simulink model "KTH_pedestrian_autoware_light_cs"  (R2019a)
settings: Solver=ode5  StartTime=0.0  StopTime=inf  FixedStep=1/20  RelTol=1e-3
PreLoadFcn:
  | mbxruntime.callbacks.PreLoadFcn(bdroot);
PostLoadFcn:
  | mbxruntime.callbacks.PostLoadFcn(bdroot);
InitFcn:
  | mbxruntime.callbacks.InitFcn(bdroot);
StartFcn:
  | mbxruntime.callbacks.StartFcn(bdroot);
StopFcn:
  | mbxruntime.callbacks.StopFcn(bdroot);
model workspace: external: MAT-File .\KTH_pedestrian_autoware_light_cs_hws.mat (data not in the file)
undefined symbols (not defined in the file or in its folder): DiscIntNeverNeededParam, KTH_pedestrian_autoware_light_cs_02ac950ed1db34ed, KTH_pedestrian_autoware_light_cs_05d7c050840f08db, KTH_pedestrian_autoware_light_cs_0ac3d38ce01e323f, KTH_pedestrian_autoware_light_cs_1214d37425b96e35, KTH_pedestrian_autoware_light_cs_2826e94662b29978, KTH_pedestrian_autoware_light_cs_284990f0f6de4093, KTH_pedestrian_autoware_light_cs_2ceb80ac95efe639, KTH_pedestrian_autoware_light_cs_5a38d8f46f118122, KTH_pedestrian_autoware_light_cs_6a647bfa7761b210, KTH_pedestrian_autoware_light_cs_790d47fa8c779a57, KTH_pedestrian_autoware_light_cs_7e2644aa1be91b53, KTH_pedestrian_autoware_light_cs_7f1596adbf6cd625, KTH_pedestrian_autoware_light_cs_8d332c892ff4a2b3, KTH_pedestrian_autoware_light_cs_a7eac5b1261ff56b, KTH_pedestrian_autoware_light_cs_b4a916664d8e8a9c, KTH_pedestrian_autoware_light_cs_ece26882e18d2248, KTH_pedestrian_autoware_light_cs_fb19b2cd0788cd5c, KTH_pedestrian_autoware_light_cs_fbb215df62dd156c, mbxruntime, tabledata, X, Y, Z
libraries: adeye_lib x16, PreScanSimulinkLibrary x6, robotlib x2, PreScanUsefulBlocks x1, simulink x1
(part 2 of 3)

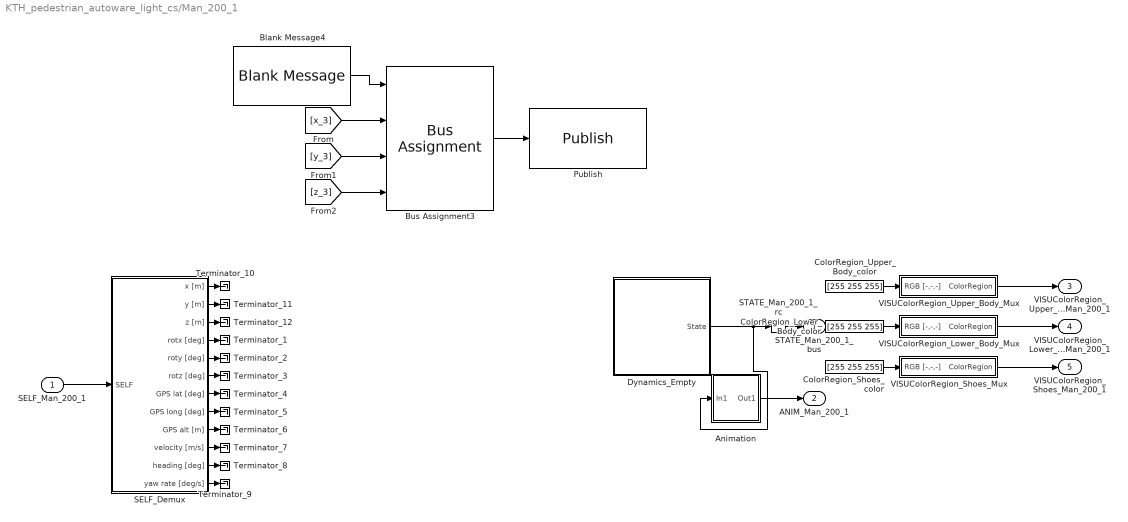
== system KTH_pedestrian_autoware_light_cs/Man_200_1 ==
  SELF_Man_200_1 : Inport  Tag=inport/SelfPort  OutDataTypeStr=Bus: PRESCAN_SELFSENSORDATA  PortDimensions=1  SampleTime=1/20  BusOutputAsStruct=on
  Animation : Subsystem  Tag=WalkingHumanAnimation  mask(Prescan Conversion Block: Walking Human Animation){TimeStep=1/20}
      mask prompts: TimeStep "Auto-Assigned: Upload Period [s]"
      mask help: The Walking Human Animation block converts the State signal of a human into signals to properly control the animation.
      mask Help: eval('openHelp(239)');
      mask Display: image(imread('HumanAnimated.jpg'))
  Blank Message4 : robotlib/Blank Message  messageClass=Message  entityType=geometry_msgs/Point  messageType=geometry_msgs/Point  SampleTime=inf
      settings: SourceProductBaseCode=RO
  Bus Assignment3 : BusAssignment  AssignedSignals=X,Y,Z
  ColorRegion_Lower_Body_color : Constant  Tag=VisuLightConst  Value=[255 255 255]
  ColorRegion_Shoes_color : Constant  Tag=VisuLightConst  Value=[255 255 255]
  ColorRegion_Upper_Body_color : Constant  Tag=VisuLightConst  Value=[255 255 255]
  Dynamics_Empty : Subsystem  Tag=Dynamics_Empty
      mask Help: eval('openHelp(202)')
      mask Display: port_label('output', 1, 'State');text(0,0,' Empty\n')
  Publish : robotlib/Publish  topicSource=Specify your own  topic=/simulink/pedestrian_pose  messageType=geometry_msgs/Point  messageQueueLength=1
      settings: SourceProductBaseCode=RO
  SELF_Demux : Subsystem  Tag=demux/SelfPort  mask(PreScan Demux Block:){}
      mask help:
      | The SELF port shows (state) information of the actor itself. The outputs are position in the experiment's axis system and the GPS coordinates, and the object's absolute velocity and compass heading.
      |
      | For more information, please click Help.
      settings: DeleteFcn=PreScanBlockDeleteFcn;
      mask Help: eval('openHelp(462)')
      mask Display:
      | port_label('output',1,'x [m]')
      | port_label('output',2,'y [m]')
      | port_label('output',3,'z [m]','texmode','on')
      | port_label('output',4,'Rotx [deg]','texmode','on')
      | port_label('output',5,'Roty [deg]','texmode','on')
      | port_label('output',6,'Rotz [deg]','texmode','on')
      | port_label('output',7,'GPS lat [deg]','texmode','on')
      | port_label('output',8,'GPS long [deg]','texmode','on')
      | port_label('output',9,'GPS alt [m]','texmode','on')
      | port_label('output',10,'Velocity [m/s]')
      | port_label('output',11,'Heading [deg]')
      | port_label('output',12,'Yaw rate [deg/s]')
  STATE_Man_200_1_rc : RateTransition  Tag=mux_rc/StatePort  OutPortSampleTimeOpt=Inherit
  Terminator_{1..12} (12 alike) : Terminator
  VISUColorRegion_Lower_Body_Mux : Subsystem  Tag=mux/MuxColorRegion  LoadFcn=load PrescanColorData  mask(PreScan User Interface: VisuTextureColor){}
      mask help:
      | The VisuTextureColor block provides a way to adapt the color of a vehicle.
      |
      | For more information, please click Help.
      settings: DeleteFcn=PreScanBlockDeleteFcn;
      mask Help: eval('openHelp(230)')
  VISUColorRegion_Shoes_Mux : Subsystem  Tag=mux/MuxColorRegion  LoadFcn=load PrescanColorData  mask(PreScan User Interface: VisuTextureColor){}
      mask help:
      | The VisuTextureColor block provides a way to adapt the color of a vehicle.
      |
      | For more information, please click Help.
      settings: DeleteFcn=PreScanBlockDeleteFcn;
      mask Help: eval('openHelp(230)')
  VISUColorRegion_Upper_Body_Mux : Subsystem  Tag=mux/MuxColorRegion  LoadFcn=load PrescanColorData  mask(PreScan User Interface: VisuTextureColor){}
      mask help:
      | The VisuTextureColor block provides a way to adapt the color of a vehicle.
      |
      | For more information, please click Help.
      settings: DeleteFcn=PreScanBlockDeleteFcn;
      mask Help: eval('openHelp(230)')
  STATE_Man_200_1_bus : Outport  Tag=outport/StatePort  OutDataTypeStr=Bus: PRESCAN_STATEACTUATORDATA  PortDimensions=1  SampleTime=1/20
  ANIM_Man_200_1 : Outport  Tag=outport/AnimationOutport  Port=2  OutDataTypeStr=Bus: PRESCAN_ANIMACTUATORDATA  PortDimensions=1  SampleTime=1/20
  VISUColorRegion_Upper_Body_Man_200_1 : Outport  Tag=outport/ColorRegion  Port=3  OutDataTypeStr=Bus: PRESCAN_COLOR_DATA  PortDimensions=1  SampleTime=1/20
  VISUColorRegion_Lower_Body_Man_200_1 : Outport  Tag=outport/ColorRegion  Port=4  OutDataTypeStr=Bus: PRESCAN_COLOR_DATA  PortDimensions=1  SampleTime=1/20
  VISUColorRegion_Shoes_Man_200_1 : Outport  Tag=outport/ColorRegion  Port=5  OutDataTypeStr=Bus: PRESCAN_COLOR_DATA  PortDimensions=1  SampleTime=1/20
  wires:
  Bus Assignment3/1 -> Publish/1
  Blank Message4/1 -> Bus Assignment3/1
  STATE_Man_200_1_rc/1 -> STATE_Man_200_1_bus/1
  Animation/1(Out1) -> ANIM_Man_200_1/1
  SELF_Man_200_1/1 -> SELF_Demux/1(SELF)
  VISUColorRegion_Upper_Body_Mux/1(ColorRegion) -> VISUColorRegion_Upper_Body_Man_200_1/1
  ColorRegion_Upper_Body_color/1 -> VISUColorRegion_Upper_Body_Mux/1(RGB [-,-,-])
  VISUColorRegion_Lower_Body_Mux/1(ColorRegion) -> VISUColorRegion_Lower_Body_Man_200_1/1
  ColorRegion_Lower_Body_color/1 -> VISUColorRegion_Lower_Body_Mux/1(RGB [-,-,-])
  VISUColorRegion_Shoes_Mux/1(ColorRegion) -> VISUColorRegion_Shoes_Man_200_1/1
  ColorRegion_Shoes_color/1 -> VISUColorRegion_Shoes_Mux/1(RGB [-,-,-])
  Dynamics_Empty/1(State) -> STATE_Man_200_1_rc/1, Animation/1(In1)
  SELF_Demux/4(rotx [deg]) -> Terminator_1/1
  SELF_Demux/5(roty [deg]) -> Terminator_2/1
  SELF_Demux/6(rotz [deg]) -> Terminator_3/1
  SELF_Demux/7(GPS lat [deg]) -> Terminator_4/1
  SELF_Demux/8(GPS long [deg]) -> Terminator_5/1
  SELF_Demux/9(GPS alt [m]) -> Terminator_6/1
  SELF_Demux/10(velocity [m/s]) -> Terminator_7/1
  SELF_Demux/11(heading [deg]) -> Terminator_8/1
  SELF_Demux/12(yaw rate [deg/s]) -> Terminator_9/1
  SELF_Demux/1(x [m]) -> Terminator_10/1
  SELF_Demux/2(y [m]) -> Terminator_11/1
  SELF_Demux/3(z [m]) -> Terminator_12/1
  [x_3] -> Bus Assignment3/2
  [y_3] -> Bus Assignment3/3
  [z_3] -> Bus Assignment3/4

== system KTH_pedestrian_autoware_light_cs/PointCloudSensor_1 ==
  Sensor : S-Function  FunctionName=sfun_PCS  Parameters=sensorID, dataWidth, dataHeight, numChannels, dataType, timestep  SFunctionDeploymentMode=off  EnableBusSupport=off  mask(PreScan Source Block: Point Cloud Sensor){sensorID=9052, dataWidth=16, dataHeight=900, numChannels=4, dataType=0, timestep=1/20}
      mask prompts: sensorID "Sensor ID"; dataWidth "Data Width"; dataHeight "Data Height"; numChannels "Channel Count"; dataType "Data Type"; timestep "MATLAB timestep:"
      mask help: The Point Cloud Sensor provides XYZ positions relative to the sensor
      mask Help: eval('openHelp(6400)')
      mask Display: image(imread('PointCloudSensorSL.png'))
  PointCloudSensor_1 : Outport  Tag=outport/PointCloudInport  OutDataTypeStr=single  SampleTime=1/20
  wires:
  Sensor/1 -> PointCloudSensor_1/1

== system KTH_pedestrian_autoware_light_cs/PointCloudSensor_2 ==
  Sensor : S-Function  FunctionName=sfun_PCS  Parameters=sensorID, dataWidth, dataHeight, numChannels, dataType, timestep  SFunctionDeploymentMode=off  EnableBusSupport=off  mask(PreScan Source Block: Point Cloud Sensor){sensorID=9053, dataWidth=16, dataHeight=900, numChannels=4, dataType=0, timestep=1/20}
      mask prompts: sensorID "Sensor ID"; dataWidth "Data Width"; dataHeight "Data Height"; numChannels "Channel Count"; dataType "Data Type"; timestep "MATLAB timestep:"
      mask help: The Point Cloud Sensor provides XYZ positions relative to the sensor
      mask Help: eval('openHelp(6400)')
      mask Display: image(imread('PointCloudSensorSL.png'))
  PointCloudSensor_2 : Outport  Tag=outport/PointCloudInport  OutDataTypeStr=single  SampleTime=1/20
  wires:
  Sensor/1 -> PointCloudSensor_2/1

== system KTH_pedestrian_autoware_light_cs/PointCloudSensor_3 ==
  Sensor : S-Function  FunctionName=sfun_PCS  Parameters=sensorID, dataWidth, dataHeight, numChannels, dataType, timestep  SFunctionDeploymentMode=off  EnableBusSupport=off  mask(PreScan Source Block: Point Cloud Sensor){sensorID=9054, dataWidth=16, dataHeight=900, numChannels=4, dataType=0, timestep=1/20}
      mask prompts: sensorID "Sensor ID"; dataWidth "Data Width"; dataHeight "Data Height"; numChannels "Channel Count"; dataType "Data Type"; timestep "MATLAB timestep:"
      mask help: The Point Cloud Sensor provides XYZ positions relative to the sensor
      mask Help: eval('openHelp(6400)')
      mask Display: image(imread('PointCloudSensorSL.png'))
  PointCloudSensor_3 : Outport  Tag=outport/PointCloudInport  OutDataTypeStr=single  SampleTime=1/20
  wires:
  Sensor/1 -> PointCloudSensor_3/1

== system KTH_pedestrian_autoware_light_cs/PointCloudSensor_4 ==
  Sensor : S-Function  FunctionName=sfun_PCS  Parameters=sensorID, dataWidth, dataHeight, numChannels, dataType, timestep  SFunctionDeploymentMode=off  EnableBusSupport=off  mask(PreScan Source Block: Point Cloud Sensor){sensorID=9055, dataWidth=16, dataHeight=900, numChannels=4, dataType=0, timestep=1/20}
      mask prompts: sensorID "Sensor ID"; dataWidth "Data Width"; dataHeight "Data Height"; numChannels "Channel Count"; dataType "Data Type"; timestep "MATLAB timestep:"
      mask help: The Point Cloud Sensor provides XYZ positions relative to the sensor
      mask Help: eval('openHelp(6400)')
      mask Display: image(imread('PointCloudSensorSL.png'))
  PointCloudSensor_4 : Outport  Tag=outport/PointCloudInport  OutDataTypeStr=single  SampleTime=1/20
  wires:
  Sensor/1 -> PointCloudSensor_4/1

== system KTH_pedestrian_autoware_light_cs/PreScanTerminator ==
  Terminator : Terminator
  sfun_Terminator : S-Function  FunctionName=sfun_Terminator  Parameters=SampleTime  SFunctionDeploymentMode=off  EnableBusSupport=off  mask(Legacy Function){SFunctionSpec=void prescan_terminator_outputFcn(void ** work1, PRESCAN_TERMINATORDATA y1[1]), SampleTime=TimeStep, ShowSpec=on}
      mask prompts: SampleTime "Sample time (-1 for inherited):"; ShowSpec "Display function specification"
      mask help:
      | This block allows you to call the legacy functions specified by the following Legacy Code Tool definition:
      | def.SFunctionName = 'sfun_Terminator';
      | def.OutputFcnSpec = 'void prescan_terminator_outputFcn(void ** work1, PRESCAN_TERMINATORDATA y1[1])';
      | def.StartFcnSpec = 'void prescan_terminator_startFcn(void ** work1)';
      | def.TerminateFcnSpec = 'void prescan_terminator_terminateFcn(void ** work1)';
      | def.HeaderFiles = {'prescan_terminator_data.h'};
      | def.HostLibFiles = {'sensorinterfaced.lib'};
      | def.IncPaths = {'src', 'C:\prescandev\vislibrary\vis\..\pimp\include\sensors\InterfaceRTW'};
      | def.SrcPaths = {'src'};
      | def.LibPaths = {'C:\\prescandev\\vislibrary_build\lib'};
      | def.SampleTime = 'parameterized';
      | def.Options.language = 'C';
      mask Help: <p>This block was generated automatically by the Legacy Code Tool. For detailed help on this tool, call<a href="matlab:legacy_code('help')"> legacy_code('help')</a>.</p>
      mask Callback ShowSpec:
      | if strcmp(get_param(gcbh, 'ShowSpec'), 'on')
      |   set_param(gcbh, 'MaskDisplay', sprintf('fprintf(''%s'');', get_param(gcbh, 'SFunctionSpec')));
      | else
      |   set_param(gcbh, 'MaskDisplay', sprintf('fprintf(''%s'');', get_param(gcbh, 'FunctionName')));
      | end
      mask Display: fprintf('void prescan_terminator_outputFcn(void ** work1, PRESCAN_TERMINATORDATA y1[1])');
  wires:
  sfun_Terminator/1 -> Terminator/1

== system KTH_pedestrian_autoware_light_cs/Radar_1 ==
  Sensor : S-Function  FunctionName=sfun_Radar  Parameters=sensorID, detectableObjects, timestep  SFunctionDeploymentMode=off  EnableBusSupport=off  mask(PreScan Source Block: Radar Sensor){sensorID=21907, detectableObjects=7, timestep=1/20}
      mask prompts: sensorID "Sensor ID"; detectableObjects "Max detectable objects:"; timestep "MATLAB timestep:"
      mask help:
      | The Radar Sensor is a detailed sensor based on a physical radar
      | model that includes Antenna GAIN Maps (AGM) and atmospheric
      | attenuation.
      |
      | For more information, please click Help.
      mask Help: eval('openHelp(1464)')
      mask Display: image(imread('Radar.png'))
  Radar_1 : Outport  Tag=outport/Radar  OutDataTypeStr=Bus: PRESCAN_SCANNERSENSOR_MESSAGE  PortDimensions=7  SampleTime=1/20
  wires:
  Sensor/1 -> Radar_1/1

== system KTH_pedestrian_autoware_light_cs/SELF_BMW_X5_SUV_1 ==
  Sensor : S-Function  FunctionName=sfun_SelfSensor  Parameters=UniqueID, TimeStep  SFunctionDeploymentMode=off  EnableBusSupport=off  mask(PreScan Source Block: SELF){UniqueID=9040, TimeStep=1/20}
      mask prompts: UniqueID "Auto-Assigned: Unique ID"; TimeStep "Auto-Assigned: Upload Period [s]"
      mask help:
      | The SELF port shows (state) information of the actor itself. The outputs are position in the experiment's axis system and the GPS coordinates, and the object's absolute velocity and compass heading.
      |
      | For more information, please click Help.
      mask Help: eval('openHelp(462)')
      mask Display: image(imread('GPS.png'))
  SELF_BMW_X5_SUV_1 : Outport  Tag=outport/SelfPort  OutDataTypeStr=Bus: PRESCAN_SELFSENSORDATA  PortDimensions=1  SampleTime=1/20
  wires:
  Sensor/1 -> SELF_BMW_X5_SUV_1/1

== system KTH_pedestrian_autoware_light_cs/SELF_KTH_3D_1 ==
  Sensor : S-Function  FunctionName=sfun_SelfSensor  Parameters=UniqueID, TimeStep  SFunctionDeploymentMode=off  EnableBusSupport=off  mask(PreScan Source Block: SELF){UniqueID=14987, TimeStep=1/20}
      mask prompts: UniqueID "Auto-Assigned: Unique ID"; TimeStep "Auto-Assigned: Upload Period [s]"
      mask help:
      | The SELF port shows (state) information of the actor itself. The outputs are position in the experiment's axis system and the GPS coordinates, and the object's absolute velocity and compass heading.
      |
      | For more information, please click Help.
      mask Help: eval('openHelp(462)')
      mask Display: image(imread('GPS.png'))
  SELF_KTH_3D_1 : Outport  Tag=outport/SelfPort  OutDataTypeStr=Bus: PRESCAN_SELFSENSORDATA  PortDimensions=1  SampleTime=1/20
  wires:
  Sensor/1 -> SELF_KTH_3D_1/1

== system KTH_pedestrian_autoware_light_cs/SELF_Man_200_1 ==
  Sensor : S-Function  FunctionName=sfun_SelfSensor  Parameters=UniqueID, TimeStep  SFunctionDeploymentMode=off  EnableBusSupport=off  mask(PreScan Source Block: SELF){UniqueID=20104, TimeStep=1/20}
      mask prompts: UniqueID "Auto-Assigned: Unique ID"; TimeStep "Auto-Assigned: Upload Period [s]"
      mask help:
      | The SELF port shows (state) information of the actor itself. The outputs are position in the experiment's axis system and the GPS coordinates, and the object's absolute velocity and compass heading.
      |
      | For more information, please click Help.
      mask Help: eval('openHelp(462)')
      mask Display: image(imread('GPS.png'))
  SELF_Man_200_1 : Outport  Tag=outport/SelfPort  OutDataTypeStr=Bus: PRESCAN_SELFSENSORDATA  PortDimensions=1  SampleTime=1/20
  wires:
  Sensor/1 -> SELF_Man_200_1/1

== system KTH_pedestrian_autoware_light_cs/STATE_BMW_X5_SUV_1_bus ==
  STATE_BMW_X5_SUV_1_bus : Inport  Tag=inport/StatePort  OutDataTypeStr=Bus: PRESCAN_STATEACTUATORDATA  PortDimensions=1  SampleTime=1/20  BusOutputAsStruct=on
  Actuator : S-Function  FunctionName=sfun_StateActuator  Parameters=UniqueID, TimeStep  SFunctionDeploymentMode=off  EnableBusSupport=off  mask(PreScan Sink Block: State){UniqueID=9040, TimeStep=1/20}
      mask prompts: UniqueID "Auto-Assigned: Unique ID"; TimeStep "Auto-Assigned: Upload Period [s]"
      mask help:
      | The Actor State contains a vector signal of size (9x1), containing the following signals:
      |
      | -  Position    	(x,y,z)             	[m]
      | -  Velocity    	(vx,vy,vz)         	[m/s]
      | -  Angles       	(Roll, Pitch, Yaw)	[rad]
      |
      | The Actor state is defined in the global axis system.
      | The state is superponed on the Initial position defined in the GUI.
      |
      | For more information, please click Help.
      mask Help: eval('openHelp(222)')
      mask Display: image(imread('State.png'))
  wires:
  STATE_BMW_X5_SUV_1_bus/1 -> Actuator/1

== system KTH_pedestrian_autoware_light_cs/STATE_KTH_3D_1_bus ==
  STATE_KTH_3D_1_bus : Inport  Tag=inport/StatePort  OutDataTypeStr=Bus: PRESCAN_STATEACTUATORDATA  PortDimensions=1  SampleTime=1/20  BusOutputAsStruct=on
  Actuator : S-Function  FunctionName=sfun_StateActuator  Parameters=UniqueID, TimeStep  SFunctionDeploymentMode=off  EnableBusSupport=off  mask(PreScan Sink Block: State){UniqueID=14987, TimeStep=1/20}
      mask prompts: UniqueID "Auto-Assigned: Unique ID"; TimeStep "Auto-Assigned: Upload Period [s]"
      mask help:
      | The Actor State contains a vector signal of size (9x1), containing the following signals:
      |
      | -  Position    	(x,y,z)             	[m]
      | -  Velocity    	(vx,vy,vz)         	[m/s]
      | -  Angles       	(Roll, Pitch, Yaw)	[rad]
      |
      | The Actor state is defined in the global axis system.
      | The state is superponed on the Initial position defined in the GUI.
      |
      | For more information, please click Help.
      mask Help: eval('openHelp(222)')
      mask Display: image(imread('State.png'))
  wires:
  STATE_KTH_3D_1_bus/1 -> Actuator/1

== system KTH_pedestrian_autoware_light_cs/STATE_Man_200_1_bus ==
  STATE_Man_200_1_bus : Inport  Tag=inport/StatePort  OutDataTypeStr=Bus: PRESCAN_STATEACTUATORDATA  PortDimensions=1  SampleTime=1/20  BusOutputAsStruct=on
  Actuator : S-Function  FunctionName=sfun_StateActuator  Parameters=UniqueID, TimeStep  SFunctionDeploymentMode=off  EnableBusSupport=off  mask(PreScan Sink Block: State){UniqueID=20104, TimeStep=1/20}
      mask prompts: UniqueID "Auto-Assigned: Unique ID"; TimeStep "Auto-Assigned: Upload Period [s]"
      mask help:
      | The Actor State contains a vector signal of size (9x1), containing the following signals:
      |
      | -  Position    	(x,y,z)             	[m]
      | -  Velocity    	(vx,vy,vz)         	[m/s]
      | -  Angles       	(Roll, Pitch, Yaw)	[rad]
      |
      | The Actor state is defined in the global axis system.
      | The state is superponed on the Initial position defined in the GUI.
      |
      | For more information, please click Help.
      mask Help: eval('openHelp(222)')
      mask Display: image(imread('State.png'))
  wires:
  STATE_Man_200_1_bus/1 -> Actuator/1

== system KTH_pedestrian_autoware_light_cs/ScenarioEngine ==
  Clock : Clock
  sfun_ScenarioEngine : S-Function  FunctionName=sfun_ScenarioEngine  Parameters=TimeStep  SFunctionDeploymentMode=off  EnableBusSupport=off
  wires:
  Clock/1 -> sfun_ScenarioEngine/1

== system KTH_pedestrian_autoware_light_cs/Synchronizer ==
  Bus Selector1 : BusSelector  OutputSignals=FederateStopped
  Stop Simulation : Stop
  sfun_Synchronizer : S-Function  FunctionName=sfun_Synchronizer  Parameters=SampleTime  SFunctionDeploymentMode=off  EnableBusSupport=off  mask(Legacy Function){SFunctionSpec=void prescan_synchronizer_outputFcn(void ** work1, PRESCAN_SYNCHRONIZEDATA y1[1]), SampleTime=TimeStep, ShowSpec=on}
      mask prompts: SampleTime "Sample time (-1 for inherited):"; ShowSpec "Display function specification"
      mask help:
      | This block allows you to call the legacy functions specified by the following Legacy Code Tool definition:
      | def.SFunctionName = 'sfun_Synchronizer';
      | def.OutputFcnSpec = 'void prescan_synchronizer_outputFcn(void ** work1, PRESCAN_SYNCHRONIZEDATA y1[1])';
      | def.StartFcnSpec = 'void prescan_synchronizer_startFcn(void ** work1)';
      | def.TerminateFcnSpec = 'void prescan_synchronizer_terminateFcn(void ** work1)';
      | def.HeaderFiles = {'prescan_synchronizer_data.h'};
      | def.HostLibFiles = {'sensorinterfaced.lib'};
      | def.IncPaths = {'src', 'C:\prescandev\vislibrary\vis\..\pimp\include\sensors\InterfaceRTW'};
      | def.SrcPaths = {'src'};
      | def.LibPaths = {'C:\\prescandev\\vislibrary_build\lib'};
      | def.SampleTime = 'parameterized';
      | def.Options.language = 'C';
      mask Help: <p>This block was generated automatically by the Legacy Code Tool. For detailed help on this tool, call<a href="matlab:legacy_code('help')"> legacy_code('help')</a>.</p>
      mask Callback ShowSpec:
      | if strcmp(get_param(gcbh, 'ShowSpec'), 'on')
      |   set_param(gcbh, 'MaskDisplay', sprintf('fprintf(''%s'');', get_param(gcbh, 'SFunctionSpec')));
      | else
      |   set_param(gcbh, 'MaskDisplay', sprintf('fprintf(''%s'');', get_param(gcbh, 'FunctionName')));
      | end
      mask Display: fprintf('void prescan_synchronizer_outputFcn(void ** work1, PRESCAN_SYNCHRONIZEDATA y1[1])');
  wires:
  Bus Selector1/1 -> Stop Simulation/1  "<FederateStopped>"
  sfun_Synchronizer/1 -> Bus Selector1/1

== system KTH_pedestrian_autoware_light_cs/VISUColorRegion_Lower_Body_Man_200_1 ==
  VISUColorRegion_Lower_Body_Man_200_1 : Inport  Tag=inport/ColorRegion  OutDataTypeStr=Bus: PRESCAN_COLOR_DATA  PortDimensions=1  SampleTime=1/20  BusOutputAsStruct=on
  Actuator : S-Function  FunctionName=sfun_ColorActuator  Parameters=mbxruntime.parameters.convert(UniqueID), mbxruntime.parameters.convert(WorldModelSubPath),tabledata, TimeStep  SFunctionDeploymentMode=off  EnableBusSupport=off  mask(PreScan Sink Block: VisuTextureColor){UniqueID=20104, WorldModelSubPath=/recolorRegion:name=Lower Body/targetColor, TimeStep=1/20}
      mask prompts: UniqueID "Parent Unique Identifier (auto-generated)"; WorldModelSubPath "WM SubPath(auto-generated)"; TimeStep "Simulink time step"
      mask help:
      | The VisuTextureColor block provides a way to adapt the color of a vehicle.
      |
      | For more information, please click Help.
      mask init:
      | [tabledata] = mbxruntime.parameters.table(UniqueID,WorldModelSubPath);
      mask Help: eval('openHelp(230)')
      mask Display: image(imread('TextureColor.png'))
  wires:
  VISUColorRegion_Lower_Body_Man_200_1/1 -> Actuator/1

== system KTH_pedestrian_autoware_light_cs/VISUColorRegion_Shoes_Man_200_1 ==
  VISUColorRegion_Shoes_Man_200_1 : Inport  Tag=inport/ColorRegion  OutDataTypeStr=Bus: PRESCAN_COLOR_DATA  PortDimensions=1  SampleTime=1/20  BusOutputAsStruct=on
  Actuator : S-Function  FunctionName=sfun_ColorActuator  Parameters=mbxruntime.parameters.convert(UniqueID), mbxruntime.parameters.convert(WorldModelSubPath),tabledata, TimeStep  SFunctionDeploymentMode=off  EnableBusSupport=off  mask(PreScan Sink Block: VisuTextureColor){UniqueID=20104, WorldModelSubPath=/recolorRegion:name=Shoes/targetColor, TimeStep=1/20}
      mask prompts: UniqueID "Parent Unique Identifier (auto-generated)"; WorldModelSubPath "WM SubPath(auto-generated)"; TimeStep "Simulink time step"
      mask help:
      | The VisuTextureColor block provides a way to adapt the color of a vehicle.
      |
      | For more information, please click Help.
      mask init:
      | [tabledata] = mbxruntime.parameters.table(UniqueID,WorldModelSubPath);
      mask Help: eval('openHelp(230)')
      mask Display: image(imread('TextureColor.png'))
  wires:
  VISUColorRegion_Shoes_Man_200_1/1 -> Actuator/1

== system KTH_pedestrian_autoware_light_cs/VISUColorRegion_Upper_Body_Man_200_1 ==
  VISUColorRegion_Upper_Body_Man_200_1 : Inport  Tag=inport/ColorRegion  OutDataTypeStr=Bus: PRESCAN_COLOR_DATA  PortDimensions=1  SampleTime=1/20  BusOutputAsStruct=on
  Actuator : S-Function  FunctionName=sfun_ColorActuator  Parameters=mbxruntime.parameters.convert(UniqueID), mbxruntime.parameters.convert(WorldModelSubPath),tabledata, TimeStep  SFunctionDeploymentMode=off  EnableBusSupport=off  mask(PreScan Sink Block: VisuTextureColor){UniqueID=20104, WorldModelSubPath=/recolorRegion:name=Upper Body/targetColor, TimeStep=1/20}
      mask prompts: UniqueID "Parent Unique Identifier (auto-generated)"; WorldModelSubPath "WM SubPath(auto-generated)"; TimeStep "Simulink time step"
      mask help:
      | The VisuTextureColor block provides a way to adapt the color of a vehicle.
      |
      | For more information, please click Help.
      mask init:
      | [tabledata] = mbxruntime.parameters.table(UniqueID,WorldModelSubPath);
      mask Help: eval('openHelp(230)')
      mask Display: image(imread('TextureColor.png'))
  wires:
  VISUColorRegion_Upper_Body_Man_200_1/1 -> Actuator/1

== system KTH_pedestrian_autoware_light_cs/BMW_X5_SUV_1/Camera_1_CM_Demux ==
  In1 : Inport
  Selector : Selector  NumberOfDimensions=2  InputPortWidth=3  IndexOptions=Index vector (dialog),Index vector (dialog)  Indices=-1,1:hres  OutputSizes=1,1
  Selector1 : Selector  NumberOfDimensions=2  InputPortWidth=3  IndexOptions=Index vector (dialog),Index vector (dialog)  Indices=-1,hres+1:hres*2  OutputSizes=1,1
  Selector2 : Selector  NumberOfDimensions=2  InputPortWidth=3  IndexOptions=Index vector (dialog),Index vector (dialog)  Indices=-1,hres*2+1:hres*3  OutputSizes=1,1
  R : Outport
  G : Outport  Port=2
  B : Outport  Port=3
  wires:
  In1/1 -> Selector1/1, Selector/1, Selector2/1
  Selector/1 -> R/1
  Selector1/1 -> G/1
  Selector2/1 -> B/1

== system KTH_pedestrian_autoware_light_cs/BMW_X5_SUV_1/Camera_2_CM_Demux ==
  In1 : Inport
  Selector : Selector  NumberOfDimensions=2  InputPortWidth=3  IndexOptions=Index vector (dialog),Index vector (dialog)  Indices=-1,1:hres  OutputSizes=1,1
  Selector1 : Selector  NumberOfDimensions=2  InputPortWidth=3  IndexOptions=Index vector (dialog),Index vector (dialog)  Indices=-1,hres+1:hres*2  OutputSizes=1,1
  Selector2 : Selector  NumberOfDimensions=2  InputPortWidth=3  IndexOptions=Index vector (dialog),Index vector (dialog)  Indices=-1,hres*2+1:hres*3  OutputSizes=1,1
  R : Outport
  G : Outport  Port=2
  B : Outport  Port=3
  wires:
  In1/1 -> Selector1/1, Selector/1, Selector2/1
  Selector/1 -> R/1
  Selector1/1 -> G/1
  Selector2/1 -> B/1

== system KTH_pedestrian_autoware_light_cs/BMW_X5_SUV_1/Camera_tl_CM_Demux ==
  In1 : Inport
  Selector : Selector  NumberOfDimensions=2  InputPortWidth=3  IndexOptions=Index vector (dialog),Index vector (dialog)  Indices=-1,1:hres  OutputSizes=1,1
  Selector1 : Selector  NumberOfDimensions=2  InputPortWidth=3  IndexOptions=Index vector (dialog),Index vector (dialog)  Indices=-1,hres+1:hres*2  OutputSizes=1,1
  Selector2 : Selector  NumberOfDimensions=2  InputPortWidth=3  IndexOptions=Index vector (dialog),Index vector (dialog)  Indices=-1,hres*2+1:hres*3  OutputSizes=1,1
  R : Outport
  G : Outport  Port=2
  B : Outport  Port=3
  wires:
  In1/1 -> Selector1/1, Selector/1, Selector2/1
  Selector/1 -> R/1
  Selector1/1 -> G/1
  Selector2/1 -> B/1

== system KTH_pedestrian_autoware_light_cs/BMW_X5_SUV_1/Dynamics_Empty ==
  note: For state mode 'Dynamic' positions
      | are not taken into account, as they
      | are computed by integrating velocity.
      | Click annotation for Help.
  Ground_{1..9} (9 alike) : Ground
  MuxState : Subsystem  Tag=mux/State  mask(Empty Dynamics State Block){positioningmode=on, TimeStep=1/20}
      mask prompts: positioningmode "Positioning Mode"; TimeStep "Auto Assigned: Time Step [s]"
      mask help:
      | Build the state of an actor based on user input.
      | The user can either use positioning mode or dynamics mode.
      | - When using positioning mode the position and orientation of the actor are set directly based on the input. Expected input is relative to the initial position and orientation of the actor. It's also possible to specify the velocity of the actor, though this input isn't used, only passed on.
      | - When using dynamics mode the position input is ignored. Expected input is velocity and orientation. The velocity is relative the current orientation of the actor, while orientation is relative to its initial orientation. The position of the actor is calculated based on the velocity and orientation given.
      settings: DeleteFcn=PreScanBlockDeleteFcn;
  STATE_BMW_X5_SUV_1 : Subsystem  Tag=mux/StatePort  Priority=0  LoadFcn=load PrescanStateActuatorData  mask(PreScan Sink Block: State){x0=KTH_pedestrian_autoware_light_cs_b4a916664d8e8a9c, y0=KTH_pedestrian_autoware_light_cs_1214d37425b96e35, z0=KTH_pedestrian_autoware_light_cs_2ceb80ac95efe639, Roll0=KTH_pedestrian_autoware_light_cs_7f1596adbf6cd625, Pitch0=KTH_pedestrian_autoware_light_cs_8d332c892ff4a2b3, Yaw0=KTH_pedestrian_autoware_light_cs_02ac950ed1db34ed, TimeStep=1/20}
      mask prompts: x0 "Ini x-position VEHICLE wrt GLOBAL axis system [m]"; y0 "Ini y-position VEHICLE wrt GLOBAL axis system [m]"; z0 "Ini z-position VEHICLE wrt GLOBAL axis system [m]"; Roll0 "Ini roll-angle BODY wrt VEHICLE axis system [deg]"; Pitch0 "Ini pitch-angle BODY wrt VEHICLE axis system [deg]"; Yaw0 "Ini yaw-angle VEHICLE wrt GLOBAL axis system [deg]"; TimeStep "Auto-Assigned: Upload Period [s]"
      mask help:
      | The Actor State contains a vector signal of size (9x1), containing the following signals:
      |
      | -  Position                  (x,y,z)                                     [m]
      | -  Velocity                  (vx,vy,vz)                               [m/s]
      | -  Angles                    (Roll, Pitch, Yaw)                   [rad]
      |
      | The Actor state is defined in the global axis system.
      | The state is superponed on the Initial position defined in the GUI.
      |
      | For more information, please click Help.
      settings: DeleteFcn=PreScanBlockDeleteFcn;
      mask Help: eval('openHelp(222)')
      mask Display: image(imread('State.png'))
  State : Outport  Tag=outport/StateOutport  SampleTime=1/20
  wires:
  MuxState/1(state) -> STATE_BMW_X5_SUV_1/1(State)
  STATE_BMW_X5_SUV_1/1(StateBus) -> State/1
  Ground_1/1 -> MuxState/1(x [m])
  Ground_2/1 -> MuxState/2(y [m])
  Ground_3/1 -> MuxState/3(z [m])
  Ground_4/1 -> MuxState/4(dx [m/s])
  Ground_5/1 -> MuxState/5(dy [m/s])
  Ground_6/1 -> MuxState/6(dz [m/s])
  Ground_7/1 -> MuxState/7(R [rad])
  Ground_8/1 -> MuxState/8(P [rad])
  Ground_9/1 -> MuxState/9(Y [rad])

== system KTH_pedestrian_autoware_light_cs/BMW_X5_SUV_1/PointCloudSensor_1_Angles_Demux ==
  In2 : Inport
  Selector : Selector  NumberOfDimensions=2  InputPortWidth=3  IndexOptions=Index vector (dialog),Index vector (dialog)  Indices=-1,offset+1:(offset+hres)  OutputSizes=1,1
  Selector1 : Selector  NumberOfDimensions=2  InputPortWidth=3  IndexOptions=Index vector (dialog),Index vector (dialog)  Indices=-1,(offset+hres+1):(offset+2*hres)  OutputSizes=1,1
  Theta : Outport
  Phi : Outport  Port=2
  wires:
  Selector1/1 -> Phi/1
  Selector/1 -> Theta/1
  In2/1 -> Selector/1, Selector1/1

== system KTH_pedestrian_autoware_light_cs/BMW_X5_SUV_1/PointCloudSensor_1_Intensity_Demux ==
  In1 : Inport
  Selector3 : Selector  NumberOfDimensions=2  InputPortWidth=3  IndexOptions=Index vector (dialog),Index vector (dialog)  Indices=-1,offset+1:(offset+hres)  OutputSizes=1,1
  Intensity : Outport
  wires:
  Selector3/1 -> Intensity/1
  In1/1 -> Selector3/1

== system KTH_pedestrian_autoware_light_cs/BMW_X5_SUV_1/PointCloudSensor_1_Range_Demux ==
  In1 : Inport
  Selector : Selector  NumberOfDimensions=2  InputPortWidth=3  IndexOptions=Index vector (dialog),Index vector (dialog)  Indices=-1,offset+1:(offset+hres)  OutputSizes=1,1
  Range : Outport
  wires:
  Selector/1 -> Range/1
  In1/1 -> Selector/1

== system KTH_pedestrian_autoware_light_cs/BMW_X5_SUV_1/PointCloudSensor_2_Angles_Demux ==
  In2 : Inport
  Selector : Selector  NumberOfDimensions=2  InputPortWidth=3  IndexOptions=Index vector (dialog),Index vector (dialog)  Indices=-1,offset+1:(offset+hres)  OutputSizes=1,1
  Selector1 : Selector  NumberOfDimensions=2  InputPortWidth=3  IndexOptions=Index vector (dialog),Index vector (dialog)  Indices=-1,(offset+hres+1):(offset+2*hres)  OutputSizes=1,1
  Theta : Outport
  Phi : Outport  Port=2
  wires:
  Selector1/1 -> Phi/1
  Selector/1 -> Theta/1
  In2/1 -> Selector/1, Selector1/1

== system KTH_pedestrian_autoware_light_cs/BMW_X5_SUV_1/PointCloudSensor_2_Intensity_Demux ==
  In1 : Inport
  Selector3 : Selector  NumberOfDimensions=2  InputPortWidth=3  IndexOptions=Index vector (dialog),Index vector (dialog)  Indices=-1,offset+1:(offset+hres)  OutputSizes=1,1
  Intensity : Outport
  wires:
  Selector3/1 -> Intensity/1
  In1/1 -> Selector3/1

== system KTH_pedestrian_autoware_light_cs/BMW_X5_SUV_1/PointCloudSensor_2_Range_Demux ==
  In1 : Inport
  Selector : Selector  NumberOfDimensions=2  InputPortWidth=3  IndexOptions=Index vector (dialog),Index vector (dialog)  Indices=-1,offset+1:(offset+hres)  OutputSizes=1,1
  Range : Outport
  wires:
  Selector/1 -> Range/1
  In1/1 -> Selector/1

== system KTH_pedestrian_autoware_light_cs/BMW_X5_SUV_1/PointCloudSensor_3_Angles_Demux ==
  In2 : Inport
  Selector : Selector  NumberOfDimensions=2  InputPortWidth=3  IndexOptions=Index vector (dialog),Index vector (dialog)  Indices=-1,offset+1:(offset+hres)  OutputSizes=1,1
  Selector1 : Selector  NumberOfDimensions=2  InputPortWidth=3  IndexOptions=Index vector (dialog),Index vector (dialog)  Indices=-1,(offset+hres+1):(offset+2*hres)  OutputSizes=1,1
  Theta : Outport
  Phi : Outport  Port=2
  wires:
  Selector1/1 -> Phi/1
  Selector/1 -> Theta/1
  In2/1 -> Selector/1, Selector1/1

== system KTH_pedestrian_autoware_light_cs/BMW_X5_SUV_1/PointCloudSensor_3_Intensity_Demux ==
  In1 : Inport
  Selector3 : Selector  NumberOfDimensions=2  InputPortWidth=3  IndexOptions=Index vector (dialog),Index vector (dialog)  Indices=-1,offset+1:(offset+hres)  OutputSizes=1,1
  Intensity : Outport
  wires:
  Selector3/1 -> Intensity/1
  In1/1 -> Selector3/1

== system KTH_pedestrian_autoware_light_cs/BMW_X5_SUV_1/PointCloudSensor_3_Range_Demux ==
  In1 : Inport
  Selector : Selector  NumberOfDimensions=2  InputPortWidth=3  IndexOptions=Index vector (dialog),Index vector (dialog)  Indices=-1,offset+1:(offset+hres)  OutputSizes=1,1
  Range : Outport
  wires:
  Selector/1 -> Range/1
  In1/1 -> Selector/1

== system KTH_pedestrian_autoware_light_cs/BMW_X5_SUV_1/PointCloudSensor_4_Angles_Demux ==
  In2 : Inport
  Selector : Selector  NumberOfDimensions=2  InputPortWidth=3  IndexOptions=Index vector (dialog),Index vector (dialog)  Indices=-1,offset+1:(offset+hres)  OutputSizes=1,1
  Selector1 : Selector  NumberOfDimensions=2  InputPortWidth=3  IndexOptions=Index vector (dialog),Index vector (dialog)  Indices=-1,(offset+hres+1):(offset+2*hres)  OutputSizes=1,1
  Theta : Outport
  Phi : Outport  Port=2
  wires:
  Selector1/1 -> Phi/1
  Selector/1 -> Theta/1
  In2/1 -> Selector/1, Selector1/1

== system KTH_pedestrian_autoware_light_cs/BMW_X5_SUV_1/PointCloudSensor_4_Intensity_Demux ==
  In1 : Inport
  Selector3 : Selector  NumberOfDimensions=2  InputPortWidth=3  IndexOptions=Index vector (dialog),Index vector (dialog)  Indices=-1,offset+1:(offset+hres)  OutputSizes=1,1
  Intensity : Outport
  wires:
  Selector3/1 -> Intensity/1
  In1/1 -> Selector3/1

== system KTH_pedestrian_autoware_light_cs/BMW_X5_SUV_1/PointCloudSensor_4_Range_Demux ==
  In1 : Inport
  Selector : Selector  NumberOfDimensions=2  InputPortWidth=3  IndexOptions=Index vector (dialog),Index vector (dialog)  Indices=-1,offset+1:(offset+hres)  OutputSizes=1,1
  Range : Outport
  wires:
  Selector/1 -> Range/1
  In1/1 -> Selector/1

== system KTH_pedestrian_autoware_light_cs/BMW_X5_SUV_1/Radar_1_Demux ==
  Radar : Inport
  Bus Selector1 : BusSelector  OutputSignals=ActiveBeamID[-],Range[m],DopplerVelocity[ms-1],DopplerVelocityX[ms-1],DopplerVelocityY[ms-1],DopplerVelocityZ[ms-1],Theta[deg],Phi[deg],TargetID[-],TargetTypeID[-],EnergyLoss[dB],Alpha[deg],Beta[deg]  OutputAsBus=on
  ScannerSensorLegacyBusConversion : PreScanUsefulBlocks/ScannerSensorLegacyBusConversion  MAXMESSAGES=MAXMESSAGES
  Radar Data : Outport
  wires:
  Bus Selector1/1 -> Radar Data/1
  ScannerSensorLegacyBusConversion/1 -> Bus Selector1/1
  Radar/1 -> ScannerSensorLegacyBusConversion/1

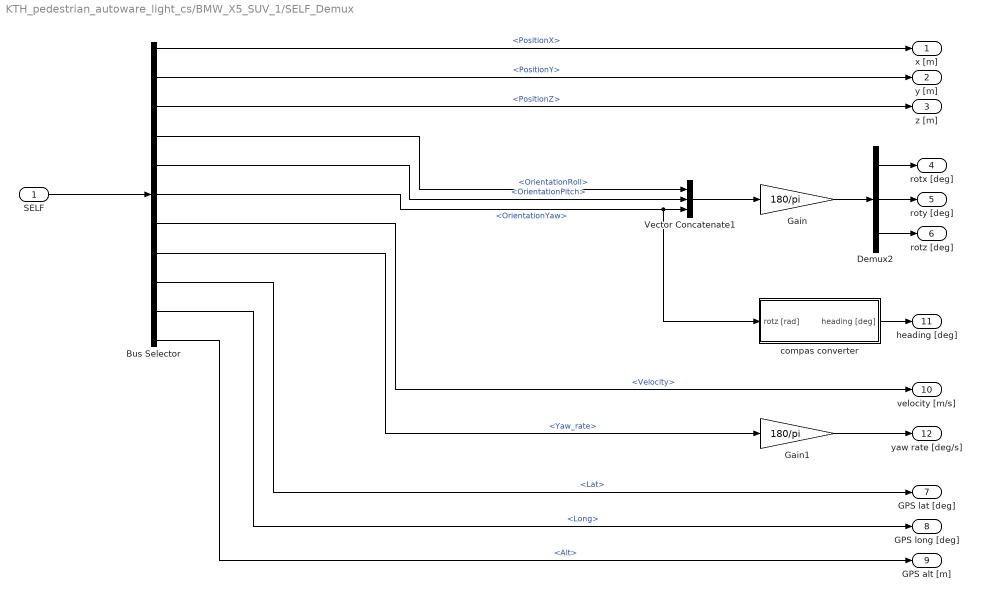
== system KTH_pedestrian_autoware_light_cs/BMW_X5_SUV_1/SELF_Demux ==
  SELF : Inport  OutDataTypeStr=Bus: PRESCAN_SELFSENSORDATA
  Bus Selector : BusSelector  OutputSignals=PositionX,PositionY,PositionZ,OrientationRoll,OrientationPitch,OrientationYaw,Velocity,Yaw_rate,Lat,Long,Alt
  Demux2 : Demux  Outputs=3
  Gain : Gain  Gain=180/pi
  Gain1 : Gain  Gain=180/pi
  Vector Concatenate1 : Concatenate  NumInputs=3
  compas converter : Subsystem
  x [m] : Outport
  y [m] : Outport  Port=2
  z [m] : Outport  Port=3
  rotx [deg] : Outport  Port=4
  roty [deg] : Outport  Port=5
  rotz [deg] : Outport  Port=6
  GPS lat [deg] : Outport  Port=7
  GPS long [deg] : Outport  Port=8
  GPS alt [m] : Outport  Port=9
  velocity [m/s] : Outport  Port=10
  heading [deg] : Outport  Port=11
  yaw rate [deg/s] : Outport  Port=12
  wires:
  Bus Selector/11 -> GPS alt [m]/1  "<Alt>"
  Bus Selector/10 -> GPS long [deg]/1  "<Long>"
  Bus Selector/9 -> GPS lat [deg]/1  "<Lat>"
  Bus Selector/8 -> Gain1/1  "<Yaw_rate>"
  Bus Selector/7 -> velocity [m/s]/1  "<Velocity>"
  Bus Selector/6 -> compas converter/1(rotz [rad]), Vector Concatenate1/3  "<OrientationYaw>"
  Bus Selector/5 -> Vector Concatenate1/2  "<OrientationPitch>"
  Bus Selector/4 -> Vector Concatenate1/1  "<OrientationRoll>"
  Vector Concatenate1/1 -> Gain/1
  Bus Selector/3 -> z [m]/1  "<PositionZ>"
  Bus Selector/2 -> y [m]/1  "<PositionY>"
  Bus Selector/1 -> x [m]/1  "<PositionX>"
  SELF/1 -> Bus Selector/1
  Gain/1 -> Demux2/1
  Demux2/1 -> rotx [deg]/1
  Demux2/2 -> roty [deg]/1
  Demux2/3 -> rotz [deg]/1
  compas converter/1(heading [deg]) -> heading [deg]/1
  Gain1/1 -> yaw rate [deg/s]/1

== system KTH_pedestrian_autoware_light_cs/KTH_3D_1/Dynamics_Empty ==
  note: For state mode 'Dynamic' positions
      | are not taken into account, as they
      | are computed by integrating velocity.
      | Click annotation for Help.
  Ground_{1..9} (9 alike) : Ground
  MuxState : Subsystem  Tag=mux/State  mask(Empty Dynamics State Block){positioningmode=on, TimeStep=1/20}
      mask prompts: positioningmode "Positioning Mode"; TimeStep "Auto Assigned: Time Step [s]"
      mask help:
      | Build the state of an actor based on user input.
      | The user can either use positioning mode or dynamics mode.
      | - When using positioning mode the position and orientation of the actor are set directly based on the input. Expected input is relative to the initial position and orientation of the actor. It's also possible to specify the velocity of the actor, though this input isn't used, only passed on.
      | - When using dynamics mode the position input is ignored. Expected input is velocity and orientation. The velocity is relative the current orientation of the actor, while orientation is relative to its initial orientation. The position of the actor is calculated based on the velocity and orientation given.
      settings: DeleteFcn=PreScanBlockDeleteFcn;
  STATE_KTH_3D_1 : Subsystem  Tag=mux/StatePort  Priority=0  LoadFcn=load PrescanStateActuatorData  mask(PreScan Sink Block: State){x0=KTH_pedestrian_autoware_light_cs_284990f0f6de4093, y0=KTH_pedestrian_autoware_light_cs_ece26882e18d2248, z0=KTH_pedestrian_autoware_light_cs_790d47fa8c779a57, Roll0=KTH_pedestrian_autoware_light_cs_5a38d8f46f118122, Pitch0=KTH_pedestrian_autoware_light_cs_6a647bfa7761b210, Yaw0=KTH_pedestrian_autoware_light_cs_7e2644aa1be91b53, TimeStep=1/20}
      mask prompts: x0 "Ini x-position VEHICLE wrt GLOBAL axis system [m]"; y0 "Ini y-position VEHICLE wrt GLOBAL axis system [m]"; z0 "Ini z-position VEHICLE wrt GLOBAL axis system [m]"; Roll0 "Ini roll-angle BODY wrt VEHICLE axis system [deg]"; Pitch0 "Ini pitch-angle BODY wrt VEHICLE axis system [deg]"; Yaw0 "Ini yaw-angle VEHICLE wrt GLOBAL axis system [deg]"; TimeStep "Auto-Assigned: Upload Period [s]"
      mask help:
      | The Actor State contains a vector signal of size (9x1), containing the following signals:
      |
      | -  Position                  (x,y,z)                                     [m]
      | -  Velocity                  (vx,vy,vz)                               [m/s]
      | -  Angles                    (Roll, Pitch, Yaw)                   [rad]
      |
      | The Actor state is defined in the global axis system.
      | The state is superponed on the Initial position defined in the GUI.
      |
      | For more information, please click Help.
      settings: DeleteFcn=PreScanBlockDeleteFcn;
      mask Help: eval('openHelp(222)')
      mask Display: image(imread('State.png'))
  State : Outport  Tag=outport/StateOutport  SampleTime=1/20
  wires:
  MuxState/1(state) -> STATE_KTH_3D_1/1(State)
  STATE_KTH_3D_1/1(StateBus) -> State/1
  Ground_1/1 -> MuxState/1(x [m])
  Ground_2/1 -> MuxState/2(y [m])
  Ground_3/1 -> MuxState/3(z [m])
  Ground_4/1 -> MuxState/4(dx [m/s])
  Ground_5/1 -> MuxState/5(dy [m/s])
  Ground_6/1 -> MuxState/6(dz [m/s])
  Ground_7/1 -> MuxState/7(R [rad])
  Ground_8/1 -> MuxState/8(P [rad])
  Ground_9/1 -> MuxState/9(Y [rad])

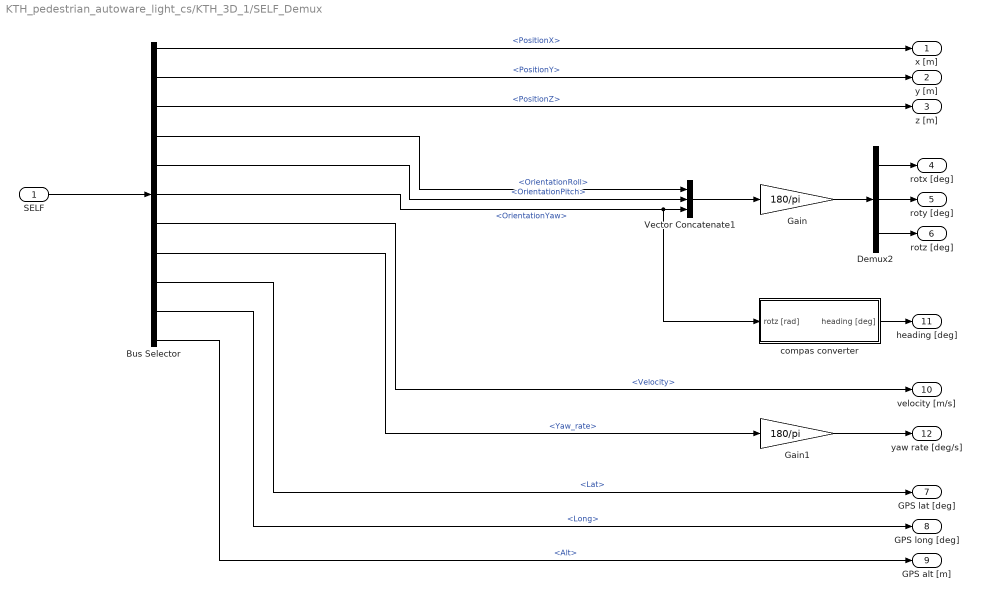
== system KTH_pedestrian_autoware_light_cs/KTH_3D_1/SELF_Demux ==
  SELF : Inport  OutDataTypeStr=Bus: PRESCAN_SELFSENSORDATA
  Bus Selector : BusSelector  OutputSignals=PositionX,PositionY,PositionZ,OrientationRoll,OrientationPitch,OrientationYaw,Velocity,Yaw_rate,Lat,Long,Alt
  Demux2 : Demux  Outputs=3
  Gain : Gain  Gain=180/pi
  Gain1 : Gain  Gain=180/pi
  Vector Concatenate1 : Concatenate  NumInputs=3
  compas converter : Subsystem
  x [m] : Outport
  y [m] : Outport  Port=2
  z [m] : Outport  Port=3
  rotx [deg] : Outport  Port=4
  roty [deg] : Outport  Port=5
  rotz [deg] : Outport  Port=6
  GPS lat [deg] : Outport  Port=7
  GPS long [deg] : Outport  Port=8
  GPS alt [m] : Outport  Port=9
  velocity [m/s] : Outport  Port=10
  heading [deg] : Outport  Port=11
  yaw rate [deg/s] : Outport  Port=12
  wires:
  Bus Selector/11 -> GPS alt [m]/1  "<Alt>"
  Bus Selector/10 -> GPS long [deg]/1  "<Long>"
  Bus Selector/9 -> GPS lat [deg]/1  "<Lat>"
  Bus Selector/8 -> Gain1/1  "<Yaw_rate>"
  Bus Selector/7 -> velocity [m/s]/1  "<Velocity>"
  Bus Selector/6 -> compas converter/1(rotz [rad]), Vector Concatenate1/3  "<OrientationYaw>"
  Bus Selector/5 -> Vector Concatenate1/2  "<OrientationPitch>"
  Bus Selector/4 -> Vector Concatenate1/1  "<OrientationRoll>"
  Vector Concatenate1/1 -> Gain/1
  Bus Selector/3 -> z [m]/1  "<PositionZ>"
  Bus Selector/2 -> y [m]/1  "<PositionY>"
  Bus Selector/1 -> x [m]/1  "<PositionX>"
  SELF/1 -> Bus Selector/1
  Gain/1 -> Demux2/1
  Demux2/1 -> rotx [deg]/1
  Demux2/2 -> roty [deg]/1
  Demux2/3 -> rotz [deg]/1
  compas converter/1(heading [deg]) -> heading [deg]/1
  Gain1/1 -> yaw rate [deg/s]/1

== system KTH_pedestrian_autoware_light_cs/Man_200_1/Animation ==
  In1 : Inport
  Bus Creator : BusCreator  Inputs=2  OutDataTypeStr=Bus: PRESCAN_ANIMACTUATORDATA  NonVirtualBus=on
  Bus Selector : BusSelector  OutputSignals=VelocityX,VelocityY,VelocityZ
  Mux : Mux  Inputs=3
  animation mode : Subsystem
  elapsed track : Subsystem
  Out1 : Outport
  wires:
  animation mode/1(mode) -> Bus Creator/1  "Index"
  Bus Creator/1 -> Out1/1
  In1/1 -> Bus Selector/1
  elapsed track/1(s) -> Bus Creator/2  "Time"
  Bus Selector/3 -> Mux/3  "<VelocityZ>"
  Bus Selector/2 -> Mux/2  "<VelocityY>"
  Bus Selector/1 -> Mux/1  "<VelocityX>"
  Mux/1 -> animation mode/1(vel), elapsed track/1(vel)

== system KTH_pedestrian_autoware_light_cs/Man_200_1/Dynamics_Empty ==
  note: For state mode 'Dynamic' positions
      | are not taken into account, as they
      | are computed by integrating velocity.
      | Click annotation for Help.
  Ground_{1..9} (9 alike) : Ground
  MuxState : Subsystem  Tag=mux/State  mask(Empty Dynamics State Block){positioningmode=on, TimeStep=1/20}
      mask prompts: positioningmode "Positioning Mode"; TimeStep "Auto Assigned: Time Step [s]"
      mask help:
      | Build the state of an actor based on user input.
      | The user can either use positioning mode or dynamics mode.
      | - When using positioning mode the position and orientation of the actor are set directly based on the input. Expected input is relative to the initial position and orientation of the actor. It's also possible to specify the velocity of the actor, though this input isn't used, only passed on.
      | - When using dynamics mode the position input is ignored. Expected input is velocity and orientation. The velocity is relative the current orientation of the actor, while orientation is relative to its initial orientation. The position of the actor is calculated based on the velocity and orientation given.
      settings: DeleteFcn=PreScanBlockDeleteFcn;
  STATE_Man_200_1 : Subsystem  Tag=mux/StatePort  Priority=0  LoadFcn=load PrescanStateActuatorData  mask(PreScan Sink Block: State){x0=KTH_pedestrian_autoware_light_cs_0ac3d38ce01e323f, y0=KTH_pedestrian_autoware_light_cs_fbb215df62dd156c, z0=KTH_pedestrian_autoware_light_cs_2826e94662b29978, Roll0=KTH_pedestrian_autoware_light_cs_05d7c050840f08db, Pitch0=KTH_pedestrian_autoware_light_cs_fb19b2cd0788cd5c, Yaw0=KTH_pedestrian_autoware_light_cs_a7eac5b1261ff56b, TimeStep=1/20}
      mask prompts: x0 "Ini x-position VEHICLE wrt GLOBAL axis system [m]"; y0 "Ini y-position VEHICLE wrt GLOBAL axis system [m]"; z0 "Ini z-position VEHICLE wrt GLOBAL axis system [m]"; Roll0 "Ini roll-angle BODY wrt VEHICLE axis system [deg]"; Pitch0 "Ini pitch-angle BODY wrt VEHICLE axis system [deg]"; Yaw0 "Ini yaw-angle VEHICLE wrt GLOBAL axis system [deg]"; TimeStep "Auto-Assigned: Upload Period [s]"
      mask help:
      | The Actor State contains a vector signal of size (9x1), containing the following signals:
      |
      | -  Position                  (x,y,z)                                     [m]
      | -  Velocity                  (vx,vy,vz)                               [m/s]
      | -  Angles                    (Roll, Pitch, Yaw)                   [rad]
      |
      | The Actor state is defined in the global axis system.
      | The state is superponed on the Initial position defined in the GUI.
      |
      | For more information, please click Help.
      settings: DeleteFcn=PreScanBlockDeleteFcn;
      mask Help: eval('openHelp(222)')
      mask Display: image(imread('State.png'))
  State : Outport  Tag=outport/StateOutport  SampleTime=1/20
  wires:
  MuxState/1(state) -> STATE_Man_200_1/1(State)
  STATE_Man_200_1/1(StateBus) -> State/1
  Ground_1/1 -> MuxState/1(x [m])
  Ground_2/1 -> MuxState/2(y [m])
  Ground_3/1 -> MuxState/3(z [m])
  Ground_4/1 -> MuxState/4(dx [m/s])
  Ground_5/1 -> MuxState/5(dy [m/s])
  Ground_6/1 -> MuxState/6(dz [m/s])
  Ground_7/1 -> MuxState/7(R [rad])
  Ground_8/1 -> MuxState/8(P [rad])
  Ground_9/1 -> MuxState/9(Y [rad])

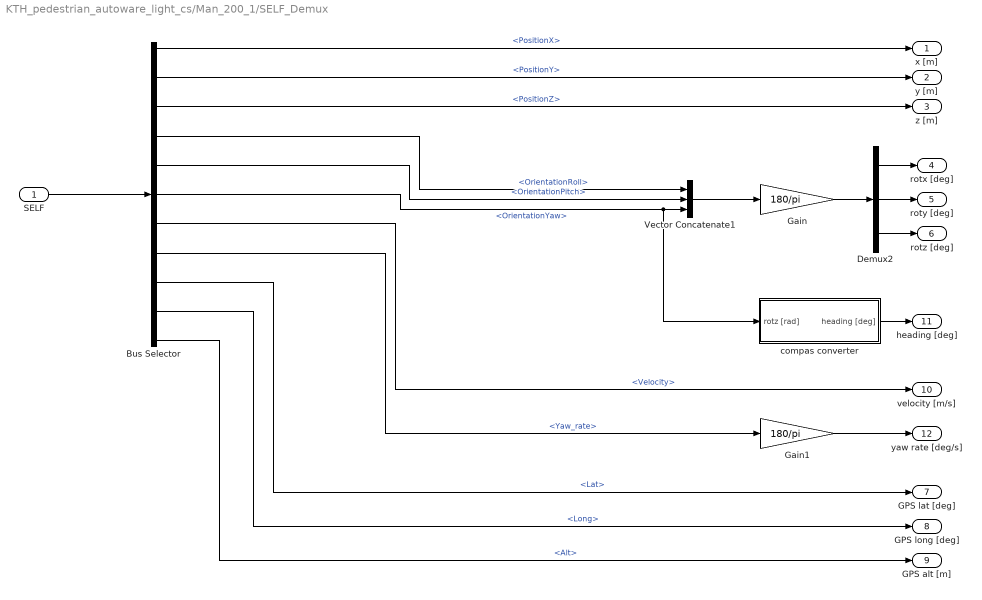
== system KTH_pedestrian_autoware_light_cs/Man_200_1/SELF_Demux ==
  SELF : Inport  OutDataTypeStr=Bus: PRESCAN_SELFSENSORDATA
  Bus Selector : BusSelector  OutputSignals=PositionX,PositionY,PositionZ,OrientationRoll,OrientationPitch,OrientationYaw,Velocity,Yaw_rate,Lat,Long,Alt
  Demux2 : Demux  Outputs=3
  Gain : Gain  Gain=180/pi
  Gain1 : Gain  Gain=180/pi
  Vector Concatenate1 : Concatenate  NumInputs=3
  compas converter : Subsystem
  x [m] : Outport
  y [m] : Outport  Port=2
  z [m] : Outport  Port=3
  rotx [deg] : Outport  Port=4
  roty [deg] : Outport  Port=5
  rotz [deg] : Outport  Port=6
  GPS lat [deg] : Outport  Port=7
  GPS long [deg] : Outport  Port=8
  GPS alt [m] : Outport  Port=9
  velocity [m/s] : Outport  Port=10
  heading [deg] : Outport  Port=11
  yaw rate [deg/s] : Outport  Port=12
  wires:
  Bus Selector/11 -> GPS alt [m]/1  "<Alt>"
  Bus Selector/10 -> GPS long [deg]/1  "<Long>"
  Bus Selector/9 -> GPS lat [deg]/1  "<Lat>"
  Bus Selector/8 -> Gain1/1  "<Yaw_rate>"
  Bus Selector/7 -> velocity [m/s]/1  "<Velocity>"
  Bus Selector/6 -> compas converter/1(rotz [rad]), Vector Concatenate1/3  "<OrientationYaw>"
  Bus Selector/5 -> Vector Concatenate1/2  "<OrientationPitch>"
  Bus Selector/4 -> Vector Concatenate1/1  "<OrientationRoll>"
  Vector Concatenate1/1 -> Gain/1
  Bus Selector/3 -> z [m]/1  "<PositionZ>"
  Bus Selector/2 -> y [m]/1  "<PositionY>"
  Bus Selector/1 -> x [m]/1  "<PositionX>"
  SELF/1 -> Bus Selector/1
  Gain/1 -> Demux2/1
  Demux2/1 -> rotx [deg]/1
  Demux2/2 -> roty [deg]/1
  Demux2/3 -> rotz [deg]/1
  compas converter/1(heading [deg]) -> heading [deg]/1
  Gain1/1 -> yaw rate [deg/s]/1

== system KTH_pedestrian_autoware_light_cs/Man_200_1/VISUColorRegion_Lower_Body_Mux ==
  RGB [-,-,-] : Inport
  Bus Creator : BusCreator  Inputs=4  OutDataTypeStr=Bus: PRESCAN_COLOR_DATA  NonVirtualBus=on
  Constant : Constant  Value=255  OutDataTypeStr=uint8
  Data Type Conversion : DataTypeConversion  OutDataTypeStr=uint8
  Data Type Conversion1 : DataTypeConversion  OutDataTypeStr=uint8
  Data Type Conversion2 : DataTypeConversion  OutDataTypeStr=uint8
  Demux : Demux  Outputs=3
  ColorRegion : Outport  OutDataTypeStr=Bus: PRESCAN_COLOR_DATA  PortDimensions=1
  wires:
  Constant/1 -> Bus Creator/4  "A"
  Data Type Conversion2/1 -> Bus Creator/3  "B"
  Data Type Conversion1/1 -> Bus Creator/2  "G"
  Data Type Conversion/1 -> Bus Creator/1  "R"
  Demux/3 -> Data Type Conversion2/1  "B"
  Demux/2 -> Data Type Conversion1/1  "G"
  Demux/1 -> Data Type Conversion/1  "R"
  RGB [-,-,-]/1 -> Demux/1
  Bus Creator/1 -> ColorRegion/1
